simulink model "disc_brake"  (R2021a)
settings: Solver=VariableStepAuto  StartTime=0.0  StopTime=5  RelTol=1e-3
settings Model: Creator=USER  LastModifiedBy=USER
settings SolverCC: AlgebraicLoopSolver=TrustRegion
settings DebuggingCC: SFMachineParentedDataDiag=warning

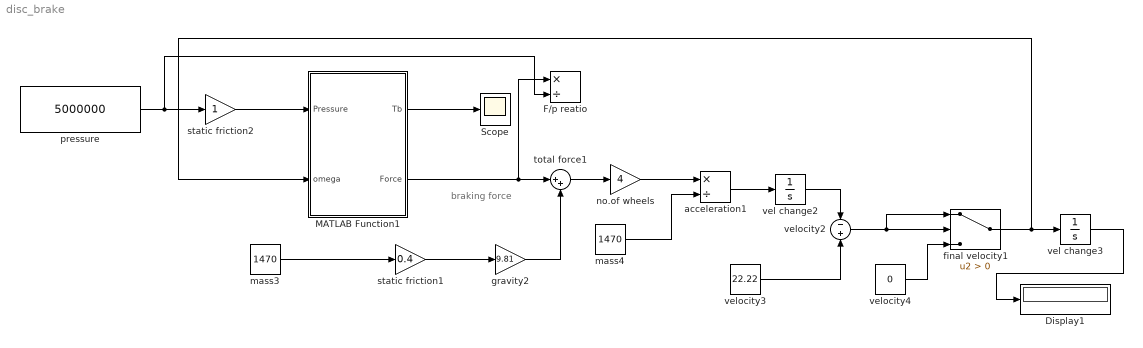
== system disc_brake ==
  note: braking force
  Display1 : Display
  F/p reatio : Product  Inputs=*/
  MATLAB Function1 : MATLAB Function  TreatAsAtomicUnit=on
  Scope : Scope
  acceleration1 : Product  Inputs=*/
  final velocity1 : Switch  Criteria=u2 > Threshold
  gravity2 : Gain  Gain=9.81
  mass3 : Constant  Value=1470  OutDataTypeStr=double
  mass4 : Constant  Value=1470
  no.of wheels : Gain  Gain=4
  pressure : Constant  Value=5000000
  static friction1 : Gain  Gain=0.4
  static friction2 : Gain
  total force1 : Sum  Inputs=|++
  vel change2 : Integrator
  vel change3 : Integrator
  velocity2 : Sum  Inputs=-+
  velocity3 : Constant  Value=22.22
  velocity4 : Constant  Value=0
  wires:
  MATLAB Function1/2(Force) -> F/p reatio/1, total force1/1
  velocity2/1 -> final velocity1/1, final velocity1/2
  no.of wheels/1 -> acceleration1/1
  velocity3/1 -> velocity2/2
  mass4/1 -> acceleration1/2
  velocity4/1 -> final velocity1/3
  static friction1/1 -> gravity2/1
  acceleration1/1 -> vel change2/1
  pressure/1 -> F/p reatio/2, static friction2/1
  mass3/1 -> static friction1/1
  gravity2/1 -> total force1/2
  vel change3/1 -> Display1/1
  vel change2/1 -> velocity2/1
  total force1/1 -> no.of wheels/1
  final velocity1/1 -> vel change3/1, MATLAB Function1/2(omega)
  MATLAB Function1/1(Tb) -> Scope/1
  static friction2/1 -> MATLAB Function1/1(Pressure)

== matlab function disc_brake/MATLAB Function1 ==
  data: Pressure input; Tb output; omega input; Force output
function [Tb,Force] = disc_brake(Pressure,omega)

% inputs to be taken
Us = 0.9;      % static friction
Uk = 0.8;     % kinetic friction       
Db = 0.09;    % brake actuator bore diameter
Rm = 0.177 ;     % mean radius of brake pad force application on brake rotor.
N_p = 2;      % number of brake pads in disc brake assembly.

T_f = (Pressure * pi * Db*Db * Rm * N_p) / 4;

if omega == 0
    Tb = Us * T_f;
    Force = Tb/Rm;
else
    Tb = Uk * T_f
    Force = Tb/Rm;
end
